simulink model "D53_LKA_Software"  (R2018b)
settings: Solver=ode3  StartTime=0.0  StopTime=10.0  FixedStep=0.01  RelTol=1e-3  EnableMultiTasking=on
model workspace (MAT data in the model file):
  MCOS : class17 (value not decoded)
  MCOS : class17 (value not decoded)
  MCOS : class17 (value not decoded)
  MCOS : class17 (value not decoded)
  MCOS : class17 (value not decoded)
  MCOS : class17 (value not decoded)
  MCOS : class17 (value not decoded)
  MCOS : class17 (value not decoded)
  MCOS : class17 (value not decoded)
  MCOS : class17 (value not decoded)
  MCOS : class17 (value not decoded)
  MCOS : class17 (value not decoded)
  MCOS : class17 (value not decoded)
  MCOS : class17 (value not decoded)
  MCOS : class17 (value not decoded)
  MCOS : class17 (value not decoded)
  MCOS : class17 (value not decoded)
  MCOS : class17 (value not decoded)
  MCOS : class17 (value not decoded)
  MCOS : class17 (value not decoded)
  MCOS : class17 (value not decoded)
  MCOS : class17 (value not decoded)
  MCOS : class17 (value not decoded)
  MCOS : class17 (value not decoded)
  MCOS : class17 (value not decoded)
  MCOS : class17 (value not decoded)
  MCOS : class17 (value not decoded)
  MCOS : class17 (value not decoded)
  MCOS : class17 (value not decoded)
  MCOS : class17 (value not decoded)
  MCOS : class17 (value not decoded)
  MCOS : class17 (value not decoded)
  MCOS : class17 (value not decoded)
  MCOS : class17 (value not decoded)
  MCOS : class17 (value not decoded)
  MCOS : class17 (value not decoded)
  MCOS : class17 (value not decoded)
  MCOS : class17 (value not decoded)
  MCOS : class17 (value not decoded)
  MCOS : class17 (value not decoded)
  MCOS : class17 (value not decoded)
  MCOS : class17 (value not decoded)
  MCOS : class17 (value not decoded)
  MCOS : class17 (value not decoded)
  MCOS : class17 (value not decoded)
  MCOS : class17 (value not decoded)
  MCOS : class17 (value not decoded)
  MCOS : class17 (value not decoded)
  MCOS : class17 (value not decoded)
  MCOS : class17 (value not decoded)
  MCOS : class17 (value not decoded)
  MCOS : class17 (value not decoded)
  MCOS : class17 (value not decoded)
  MCOS : class17 (value not decoded)
  MCOS : class17 (value not decoded)
  MCOS : class17 (value not decoded)
  MCOS : class17 (value not decoded)
  MCOS : class17 (value not decoded)
  MCOS : class17 (value not decoded)
  MCOS : class17 (value not decoded)
  MCOS : class17 (value not decoded)
  MCOS : class17 (value not decoded)
  MCOS : class17 (value not decoded)
  MCOS : class17 (value not decoded)
  MCOS : class17 (value not decoded)
  MCOS : class17 (value not decoded)
  MCOS : class17 (value not decoded)
  MCOS : class17 (value not decoded)
  MCOS : class17 (value not decoded)
  MCOS : class17 (value not decoded)
  MCOS : class17 (value not decoded)
  MCOS : class17 (value not decoded)
  MCOS : class17 (value not decoded)
  MCOS : class17 (value not decoded)
  MCOS : class17 (value not decoded)
  MCOS : class17 (value not decoded)
  MCOS : class17 (value not decoded)
  MCOS : class17 (value not decoded)
  MCOS : class17 (value not decoded)
  MCOS : class17 (value not decoded)
  MCOS : class17 (value not decoded)
  MCOS : class17 (value not decoded)
  MCOS : class17 (value not decoded)
  MCOS : class17 (value not decoded)
  MCOS : class17 (value not decoded)
  MCOS : class17 (value not decoded)
  MCOS : class17 (value not decoded)
  MCOS : class17 (value not decoded)
  MCOS : class17 (value not decoded)
undefined symbols (not defined in the file or in its folder): LKA_CarWidth, LKA_SampleTime, LKA_StrRatio_C, LKA_Veh2CamL_C, LKA_Veh2CamW_C, LKA_WhlBaseL_C, LL_CompSWA_C, LL_CrvtPrvwT_C, LL_DesDvt_C, LL_DvtComp_C, LL_DvtPrvwT_C, LL_DvtSpdDet_vDvtSpdMin_C, LL_HdAgExT_C, LL_HdAgPrvwT_C, LL_LAccMax_C, LL_LAccRMax_C, LL_LDW_EarliestWarnLine_C, LL_LDW_LatestWarnLine_C, LL_LDWS_SUPPRESS_HEADING, LL_LFClb_TFC_DiffCtlBalance, LL_LFClb_TFC_DiffCtrlMaxSWA, LL_LFClb_TFC_DiffCtrlRatio, LL_LFClb_TFC_facmGainLutGain1_C, LL_LFClb_TFC_facmGainLutGain2_C, LL_LFClb_TFC_facmIntegRatio, LL_LFClb_TFC_facmKlat_C, LL_LFClb_TFC_FfCtlRatio_C, LL_LFClb_TFC_phiIntegCtlMaxSWA_C, LL_LFClb_TFC_tiKlatPrvwT_C, LL_LFClb_TFC_vGainLutVehSpdLwr_C, LL_LFClb_TFC_vGainLutVehSpdUpr_C, LL_LKA_EarliestWarnLine_C, LL_LKA_LatestWarnLine_C, LL_LKAExPrcs_ExitC0Dvt, LL_LKAExPrcs_ExitC0Swt, LL_LKAExPrcs_tiExitTime1, LL_LKAExPrcs_tiExitTime2, LL_LKAExPrcs_tiExitTime3, LL_LKAS_OUT_OF_CONTROL_LAT_VEL, LL_LKAS_OUT_OF_CONTROL_TTLC, LL_LKASWASyn_M0, LL_LKASWASyn_M1, LL_LKASWASyn_M2, LL_LKASWASyn_M3K, LL_LKASWASyn_SWAaddMax, LL_LKASWASyn_T2, LL_LKASWASyn_tiTrqSwaRtTime, LL_LKASWASyn_tiTrqSwaTime, LL_LKASWASyn_TrqMax, LL_LKASWASyn_TrqSwaAddSwt, LL_LKASWASyn_TrqSwaRateDiff, LL_LSpdCompT_C, LL_lStpLngth_C, LL_MAX_DELAY_EPSSTAR_TIME, LL_MAX_DRIVER_TORQUE_DISABLE, LL_MAX_DRIVER_TORQUE_ENABLE, LL_MAX_LANE_WIDTH_DISABLE, LL_MAX_LANE_WIDTH_ENABLE, LL_MAX_LAT_ACC_DISABLE, LL_MAX_LAT_ACC_ENABLE ... (+30)
libraries: simulink x167, canmsglib x52, dspstat3 x3, simulink_extras x1
(part 20 of 21)

== system D53_LKA_Software/SignalBusCreator/Body Electric System State Receive and Processing (BESRx)/Steering Lamp CAN Frame PreProcess (StLampCANFrmPPrcs)/CAN Diagnosis (CANDia)/CheckSum Diagnosis (ChkSumDia)/Bit Check(BChk)/Bit Operating (BOp)/ChksumPre7 ==
  In1 : Inport
  Data Type Conversion8 : DataTypeConversion  OutDataTypeStr=uint16
  Extract Bits1 : simulink/Logic and Bit Operations/Extract Bits  bitsToExtract=Range of bits  numBits=8  bitIdxRange=7  outScalingMode=Treat bit field as an integer
      settings: SourceProductName=Simulink
  Out1 : Outport
  wires:
  Data Type Conversion8/1 -> Out1/1
  In1/1 -> Extract Bits1/1
  Extract Bits1/1 -> Data Type Conversion8/1

== system D53_LKA_Software/SignalBusCreator/Function Keys State Receive and Processing (FKeyStRx)/Key Enable CAN Frame PreProcess (KeyEnaCANFrmPPrcs)/CAN Diagnosis (CANDia)/CheckSum Diagnosis (ChkSumDia)/Bit Check(BChk)/Bit Operating (BOp)/ChksumPre1 ==
  In1 : Inport
  Data Type Conversion7 : DataTypeConversion  OutDataTypeStr=uint16
  Out1 : Outport
  wires:
  Data Type Conversion7/1 -> Out1/1
  In1/1 -> Data Type Conversion7/1

== system D53_LKA_Software/SignalBusCreator/Function Keys State Receive and Processing (FKeyStRx)/Key Enable CAN Frame PreProcess (KeyEnaCANFrmPPrcs)/CAN Diagnosis (CANDia)/CheckSum Diagnosis (ChkSumDia)/Bit Check(BChk)/Bit Operating (BOp)/ChksumPre2 ==
  In1 : Inport
  Data Type Conversion7 : DataTypeConversion  OutDataTypeStr=uint16
  Extract Bits : simulink/Logic and Bit Operations/Extract Bits  bitsToExtract=Range of bits  numBits=8  bitIdxRange=6  outScalingMode=Treat bit field as an integer
      settings: SourceProductName=Simulink
  Out1 : Outport
  wires:
  Extract Bits/1 -> Data Type Conversion7/1
  In1/1 -> Extract Bits/1
  Data Type Conversion7/1 -> Out1/1

== system D53_LKA_Software/SignalBusCreator/Function Keys State Receive and Processing (FKeyStRx)/Key Enable CAN Frame PreProcess (KeyEnaCANFrmPPrcs)/CAN Diagnosis (CANDia)/CheckSum Diagnosis (ChkSumDia)/Bit Check(BChk)/Bit Operating (BOp)/ChksumPre3 ==
  In1 : Inport
  Data Type Conversion8 : DataTypeConversion  OutDataTypeStr=uint16
  Extract Bits1 : simulink/Logic and Bit Operations/Extract Bits  bitsToExtract=Range of bits  numBits=8  bitIdxRange=5  outScalingMode=Treat bit field as an integer
      settings: SourceProductName=Simulink
  Out1 : Outport
  wires:
  Extract Bits1/1 -> Data Type Conversion8/1
  In1/1 -> Extract Bits1/1
  Data Type Conversion8/1 -> Out1/1

== system D53_LKA_Software/SignalBusCreator/Function Keys State Receive and Processing (FKeyStRx)/Key Enable CAN Frame PreProcess (KeyEnaCANFrmPPrcs)/CAN Diagnosis (CANDia)/CheckSum Diagnosis (ChkSumDia)/Bit Check(BChk)/Bit Operating (BOp)/ChksumPre4 ==
  In1 : Inport
  Data Type Conversion8 : DataTypeConversion  OutDataTypeStr=uint16
  Extract Bits1 : simulink/Logic and Bit Operations/Extract Bits  bitsToExtract=Range of bits  numBits=8  bitIdxRange=4  outScalingMode=Treat bit field as an integer
      settings: SourceProductName=Simulink
  Out1 : Outport
  wires:
  Data Type Conversion8/1 -> Out1/1
  In1/1 -> Extract Bits1/1
  Extract Bits1/1 -> Data Type Conversion8/1

== system D53_LKA_Software/SignalBusCreator/Function Keys State Receive and Processing (FKeyStRx)/Key Enable CAN Frame PreProcess (KeyEnaCANFrmPPrcs)/CAN Diagnosis (CANDia)/CheckSum Diagnosis (ChkSumDia)/Bit Check(BChk)/Bit Operating (BOp)/ChksumPre5 ==
  In1 : Inport
  In2 : Inport  Port=2
  Add : Sum
  Data Type Conversion1 : DataTypeConversion  OutDataTypeStr=uint16
  Data Type Conversion4 : DataTypeConversion  OutDataTypeStr=uint16
  Shift Arithmetic2 : ArithShift  BitShiftNumber=-8
  Out1 : Outport
  wires:
  Data Type Conversion1/1 -> Add/2
  Data Type Conversion4/1 -> Shift Arithmetic2/1
  Add/1 -> Out1/1
  Shift Arithmetic2/1 -> Add/1
  In2/1 -> Data Type Conversion1/1
  In1/1 -> Data Type Conversion4/1

== system D53_LKA_Software/SignalBusCreator/Function Keys State Receive and Processing (FKeyStRx)/Key Enable CAN Frame PreProcess (KeyEnaCANFrmPPrcs)/CAN Diagnosis (CANDia)/CheckSum Diagnosis (ChkSumDia)/Bit Check(BChk)/Bit Operating (BOp)/ChksumPre6 ==
  In1 : Inport
  In2 : Inport  Port=2
  Add : Sum
  Data Type Conversion1 : DataTypeConversion  OutDataTypeStr=uint16
  Data Type Conversion4 : DataTypeConversion  OutDataTypeStr=uint16
  Shift Arithmetic2 : ArithShift  BitShiftNumber=-8
  Out1 : Outport
  wires:
  In1/1 -> Data Type Conversion4/1
  In2/1 -> Data Type Conversion1/1
  Shift Arithmetic2/1 -> Add/1
  Add/1 -> Out1/1
  Data Type Conversion4/1 -> Shift Arithmetic2/1
  Data Type Conversion1/1 -> Add/2

== system D53_LKA_Software/SignalBusCreator/Function Keys State Receive and Processing (FKeyStRx)/Key Enable CAN Frame PreProcess (KeyEnaCANFrmPPrcs)/CAN Diagnosis (CANDia)/CheckSum Diagnosis (ChkSumDia)/Bit Check(BChk)/Bit Operating (BOp)/ChksumPre7 ==
  In1 : Inport
  Data Type Conversion8 : DataTypeConversion  OutDataTypeStr=uint16
  Extract Bits1 : simulink/Logic and Bit Operations/Extract Bits  bitsToExtract=Range of bits  numBits=8  bitIdxRange=7  outScalingMode=Treat bit field as an integer
      settings: SourceProductName=Simulink
  Out1 : Outport
  wires:
  Extract Bits1/1 -> Data Type Conversion8/1
  In1/1 -> Extract Bits1/1
  Data Type Conversion8/1 -> Out1/1

== system D53_LKA_Software/SignalBusCreator/Lanes Information Receive and Processing (LaneRx)/L0 Information (L0Info) /CAN Diagnosis (CANDia)/CheckSum Diagnosis (ChkSumDia)/Bit Check(BChk)/Bit Operating (BOp)/ChksumPre1 ==
  In1 : Inport
  Data Type Conversion7 : DataTypeConversion  OutDataTypeStr=uint16
  Out1 : Outport
  wires:
  In1/1 -> Data Type Conversion7/1
  Data Type Conversion7/1 -> Out1/1

== system D53_LKA_Software/SignalBusCreator/Lanes Information Receive and Processing (LaneRx)/L0 Information (L0Info) /CAN Diagnosis (CANDia)/CheckSum Diagnosis (ChkSumDia)/Bit Check(BChk)/Bit Operating (BOp)/ChksumPre2 ==
  In1 : Inport
  Data Type Conversion7 : DataTypeConversion  OutDataTypeStr=uint16
  Extract Bits : simulink/Logic and Bit Operations/Extract Bits  bitsToExtract=Range of bits  numBits=8  bitIdxRange=6  outScalingMode=Treat bit field as an integer
      settings: SourceProductName=Simulink
  Out1 : Outport
  wires:
  Data Type Conversion7/1 -> Out1/1
  In1/1 -> Extract Bits/1
  Extract Bits/1 -> Data Type Conversion7/1

== system D53_LKA_Software/SignalBusCreator/Lanes Information Receive and Processing (LaneRx)/L0 Information (L0Info) /CAN Diagnosis (CANDia)/CheckSum Diagnosis (ChkSumDia)/Bit Check(BChk)/Bit Operating (BOp)/ChksumPre3 ==
  In1 : Inport
  Data Type Conversion8 : DataTypeConversion  OutDataTypeStr=uint16
  Extract Bits1 : simulink/Logic and Bit Operations/Extract Bits  bitsToExtract=Range of bits  numBits=8  bitIdxRange=5  outScalingMode=Treat bit field as an integer
      settings: SourceProductName=Simulink
  Out1 : Outport
  wires:
  Data Type Conversion8/1 -> Out1/1
  In1/1 -> Extract Bits1/1
  Extract Bits1/1 -> Data Type Conversion8/1

== system D53_LKA_Software/SignalBusCreator/Lanes Information Receive and Processing (LaneRx)/L0 Information (L0Info) /CAN Diagnosis (CANDia)/CheckSum Diagnosis (ChkSumDia)/Bit Check(BChk)/Bit Operating (BOp)/ChksumPre4 ==
  In1 : Inport
  Data Type Conversion8 : DataTypeConversion  OutDataTypeStr=uint16
  Extract Bits1 : simulink/Logic and Bit Operations/Extract Bits  bitsToExtract=Range of bits  numBits=8  bitIdxRange=4  outScalingMode=Treat bit field as an integer
      settings: SourceProductName=Simulink
  Out1 : Outport
  wires:
  Extract Bits1/1 -> Data Type Conversion8/1
  In1/1 -> Extract Bits1/1
  Data Type Conversion8/1 -> Out1/1

== system D53_LKA_Software/SignalBusCreator/Lanes Information Receive and Processing (LaneRx)/L0 Information (L0Info) /CAN Diagnosis (CANDia)/CheckSum Diagnosis (ChkSumDia)/Bit Check(BChk)/Bit Operating (BOp)/ChksumPre5 ==
  In1 : Inport
  In2 : Inport  Port=2
  Add : Sum
  Data Type Conversion1 : DataTypeConversion  OutDataTypeStr=uint16
  Data Type Conversion4 : DataTypeConversion  OutDataTypeStr=uint16
  Shift Arithmetic2 : ArithShift  BitShiftNumber=-8
  Out1 : Outport
  wires:
  In1/1 -> Data Type Conversion4/1
  In2/1 -> Data Type Conversion1/1
  Shift Arithmetic2/1 -> Add/1
  Add/1 -> Out1/1
  Data Type Conversion4/1 -> Shift Arithmetic2/1
  Data Type Conversion1/1 -> Add/2

== system D53_LKA_Software/SignalBusCreator/Lanes Information Receive and Processing (LaneRx)/L0 Information (L0Info) /CAN Diagnosis (CANDia)/CheckSum Diagnosis (ChkSumDia)/Bit Check(BChk)/Bit Operating (BOp)/ChksumPre6 ==
  In1 : Inport
  In2 : Inport  Port=2
  Add : Sum
  Data Type Conversion1 : DataTypeConversion  OutDataTypeStr=uint16
  Data Type Conversion4 : DataTypeConversion  OutDataTypeStr=uint16
  Shift Arithmetic2 : ArithShift  BitShiftNumber=-8
  Out1 : Outport
  wires:
  Data Type Conversion1/1 -> Add/2
  Data Type Conversion4/1 -> Shift Arithmetic2/1
  Add/1 -> Out1/1
  Shift Arithmetic2/1 -> Add/1
  In2/1 -> Data Type Conversion1/1
  In1/1 -> Data Type Conversion4/1

== system D53_LKA_Software/SignalBusCreator/Lanes Information Receive and Processing (LaneRx)/L0 Information (L0Info) /CAN Diagnosis (CANDia)/CheckSum Diagnosis (ChkSumDia)/Bit Check(BChk)/Bit Operating (BOp)/ChksumPre7 ==
  In1 : Inport
  Data Type Conversion8 : DataTypeConversion  OutDataTypeStr=uint16
  Extract Bits1 : simulink/Logic and Bit Operations/Extract Bits  bitsToExtract=Range of bits  numBits=8  bitIdxRange=7  outScalingMode=Treat bit field as an integer
      settings: SourceProductName=Simulink
  Out1 : Outport
  wires:
  Data Type Conversion8/1 -> Out1/1
  In1/1 -> Extract Bits1/1
  Extract Bits1/1 -> Data Type Conversion8/1

== system D53_LKA_Software/SignalBusCreator/Lanes Information Receive and Processing (LaneRx)/L1 Information (L1Info)/CAN Diagnosis (CANDia)/CheckSum Diagnosis (ChkSumDia)/Bit Check(BChk)/Bit Operating (BOp)/ChksumPre1 ==
  In1 : Inport
  Data Type Conversion7 : DataTypeConversion  OutDataTypeStr=uint16
  Out1 : Outport
  wires:
  Data Type Conversion7/1 -> Out1/1
  In1/1 -> Data Type Conversion7/1

== system D53_LKA_Software/SignalBusCreator/Lanes Information Receive and Processing (LaneRx)/L1 Information (L1Info)/CAN Diagnosis (CANDia)/CheckSum Diagnosis (ChkSumDia)/Bit Check(BChk)/Bit Operating (BOp)/ChksumPre2 ==
  In1 : Inport
  Data Type Conversion7 : DataTypeConversion  OutDataTypeStr=uint16
  Extract Bits : simulink/Logic and Bit Operations/Extract Bits  bitsToExtract=Range of bits  numBits=8  bitIdxRange=6  outScalingMode=Treat bit field as an integer
      settings: SourceProductName=Simulink
  Out1 : Outport
  wires:
  Extract Bits/1 -> Data Type Conversion7/1
  In1/1 -> Extract Bits/1
  Data Type Conversion7/1 -> Out1/1

== system D53_LKA_Software/SignalBusCreator/Lanes Information Receive and Processing (LaneRx)/L1 Information (L1Info)/CAN Diagnosis (CANDia)/CheckSum Diagnosis (ChkSumDia)/Bit Check(BChk)/Bit Operating (BOp)/ChksumPre3 ==
  In1 : Inport
  Data Type Conversion8 : DataTypeConversion  OutDataTypeStr=uint16
  Extract Bits1 : simulink/Logic and Bit Operations/Extract Bits  bitsToExtract=Range of bits  numBits=8  bitIdxRange=5  outScalingMode=Treat bit field as an integer
      settings: SourceProductName=Simulink
  Out1 : Outport
  wires:
  Extract Bits1/1 -> Data Type Conversion8/1
  In1/1 -> Extract Bits1/1
  Data Type Conversion8/1 -> Out1/1

== system D53_LKA_Software/SignalBusCreator/Lanes Information Receive and Processing (LaneRx)/L1 Information (L1Info)/CAN Diagnosis (CANDia)/CheckSum Diagnosis (ChkSumDia)/Bit Check(BChk)/Bit Operating (BOp)/ChksumPre4 ==
  In1 : Inport
  Data Type Conversion8 : DataTypeConversion  OutDataTypeStr=uint16
  Extract Bits1 : simulink/Logic and Bit Operations/Extract Bits  bitsToExtract=Range of bits  numBits=8  bitIdxRange=4  outScalingMode=Treat bit field as an integer
      settings: SourceProductName=Simulink
  Out1 : Outport
  wires:
  Data Type Conversion8/1 -> Out1/1
  In1/1 -> Extract Bits1/1
  Extract Bits1/1 -> Data Type Conversion8/1

== system D53_LKA_Software/SignalBusCreator/Lanes Information Receive and Processing (LaneRx)/L1 Information (L1Info)/CAN Diagnosis (CANDia)/CheckSum Diagnosis (ChkSumDia)/Bit Check(BChk)/Bit Operating (BOp)/ChksumPre5 ==
  In1 : Inport
  In2 : Inport  Port=2
  Add : Sum
  Data Type Conversion1 : DataTypeConversion  OutDataTypeStr=uint16
  Data Type Conversion4 : DataTypeConversion  OutDataTypeStr=uint16
  Shift Arithmetic2 : ArithShift  BitShiftNumber=-8
  Out1 : Outport
  wires:
  Data Type Conversion1/1 -> Add/2
  Data Type Conversion4/1 -> Shift Arithmetic2/1
  Add/1 -> Out1/1
  Shift Arithmetic2/1 -> Add/1
  In2/1 -> Data Type Conversion1/1
  In1/1 -> Data Type Conversion4/1

== system D53_LKA_Software/SignalBusCreator/Lanes Information Receive and Processing (LaneRx)/L1 Information (L1Info)/CAN Diagnosis (CANDia)/CheckSum Diagnosis (ChkSumDia)/Bit Check(BChk)/Bit Operating (BOp)/ChksumPre6 ==
  In1 : Inport
  In2 : Inport  Port=2
  Add : Sum
  Data Type Conversion1 : DataTypeConversion  OutDataTypeStr=uint16
  Data Type Conversion4 : DataTypeConversion  OutDataTypeStr=uint16
  Shift Arithmetic2 : ArithShift  BitShiftNumber=-8
  Out1 : Outport
  wires:
  In1/1 -> Data Type Conversion4/1
  In2/1 -> Data Type Conversion1/1
  Shift Arithmetic2/1 -> Add/1
  Add/1 -> Out1/1
  Data Type Conversion4/1 -> Shift Arithmetic2/1
  Data Type Conversion1/1 -> Add/2

== system D53_LKA_Software/SignalBusCreator/Lanes Information Receive and Processing (LaneRx)/L1 Information (L1Info)/CAN Diagnosis (CANDia)/CheckSum Diagnosis (ChkSumDia)/Bit Check(BChk)/Bit Operating (BOp)/ChksumPre7 ==
  In1 : Inport
  Data Type Conversion8 : DataTypeConversion  OutDataTypeStr=uint16
  Extract Bits1 : simulink/Logic and Bit Operations/Extract Bits  bitsToExtract=Range of bits  numBits=8  bitIdxRange=7  outScalingMode=Treat bit field as an integer
      settings: SourceProductName=Simulink
  Out1 : Outport
  wires:
  Extract Bits1/1 -> Data Type Conversion8/1
  In1/1 -> Extract Bits1/1
  Data Type Conversion8/1 -> Out1/1

== system D53_LKA_Software/SignalBusCreator/Lanes Information Receive and Processing (LaneRx)/R0 Information (R0Info)/CAN Diagnosis (CANDia)/CheckSum Diagnosis (ChkSumDia)/Bit Check(BChk)/Bit Operating (BOp)/ChksumPre1 ==
  In1 : Inport
  Data Type Conversion7 : DataTypeConversion  OutDataTypeStr=uint16
  Out1 : Outport
  wires:
  Data Type Conversion7/1 -> Out1/1
  In1/1 -> Data Type Conversion7/1

== system D53_LKA_Software/SignalBusCreator/Lanes Information Receive and Processing (LaneRx)/R0 Information (R0Info)/CAN Diagnosis (CANDia)/CheckSum Diagnosis (ChkSumDia)/Bit Check(BChk)/Bit Operating (BOp)/ChksumPre2 ==
  In1 : Inport
  Data Type Conversion7 : DataTypeConversion  OutDataTypeStr=uint16
  Extract Bits : simulink/Logic and Bit Operations/Extract Bits  bitsToExtract=Range of bits  numBits=8  bitIdxRange=6  outScalingMode=Treat bit field as an integer
      settings: SourceProductName=Simulink
  Out1 : Outport
  wires:
  Extract Bits/1 -> Data Type Conversion7/1
  In1/1 -> Extract Bits/1
  Data Type Conversion7/1 -> Out1/1

== system D53_LKA_Software/SignalBusCreator/Lanes Information Receive and Processing (LaneRx)/R0 Information (R0Info)/CAN Diagnosis (CANDia)/CheckSum Diagnosis (ChkSumDia)/Bit Check(BChk)/Bit Operating (BOp)/ChksumPre3 ==
  In1 : Inport
  Data Type Conversion8 : DataTypeConversion  OutDataTypeStr=uint16
  Extract Bits1 : simulink/Logic and Bit Operations/Extract Bits  bitsToExtract=Range of bits  numBits=8  bitIdxRange=5  outScalingMode=Treat bit field as an integer
      settings: SourceProductName=Simulink
  Out1 : Outport
  wires:
  Extract Bits1/1 -> Data Type Conversion8/1
  In1/1 -> Extract Bits1/1
  Data Type Conversion8/1 -> Out1/1

== system D53_LKA_Software/SignalBusCreator/Lanes Information Receive and Processing (LaneRx)/R0 Information (R0Info)/CAN Diagnosis (CANDia)/CheckSum Diagnosis (ChkSumDia)/Bit Check(BChk)/Bit Operating (BOp)/ChksumPre4 ==
  In1 : Inport
  Data Type Conversion8 : DataTypeConversion  OutDataTypeStr=uint16
  Extract Bits1 : simulink/Logic and Bit Operations/Extract Bits  bitsToExtract=Range of bits  numBits=8  bitIdxRange=4  outScalingMode=Treat bit field as an integer
      settings: SourceProductName=Simulink
  Out1 : Outport
  wires:
  Data Type Conversion8/1 -> Out1/1
  In1/1 -> Extract Bits1/1
  Extract Bits1/1 -> Data Type Conversion8/1

== system D53_LKA_Software/SignalBusCreator/Lanes Information Receive and Processing (LaneRx)/R0 Information (R0Info)/CAN Diagnosis (CANDia)/CheckSum Diagnosis (ChkSumDia)/Bit Check(BChk)/Bit Operating (BOp)/ChksumPre5 ==
  In1 : Inport
  In2 : Inport  Port=2
  Add : Sum
  Data Type Conversion1 : DataTypeConversion  OutDataTypeStr=uint16
  Data Type Conversion4 : DataTypeConversion  OutDataTypeStr=uint16
  Shift Arithmetic2 : ArithShift  BitShiftNumber=-8
  Out1 : Outport
  wires:
  Data Type Conversion1/1 -> Add/2
  Data Type Conversion4/1 -> Shift Arithmetic2/1
  Add/1 -> Out1/1
  Shift Arithmetic2/1 -> Add/1
  In2/1 -> Data Type Conversion1/1
  In1/1 -> Data Type Conversion4/1

== system D53_LKA_Software/SignalBusCreator/Lanes Information Receive and Processing (LaneRx)/R0 Information (R0Info)/CAN Diagnosis (CANDia)/CheckSum Diagnosis (ChkSumDia)/Bit Check(BChk)/Bit Operating (BOp)/ChksumPre6 ==
  In1 : Inport
  In2 : Inport  Port=2
  Add : Sum
  Data Type Conversion1 : DataTypeConversion  OutDataTypeStr=uint16
  Data Type Conversion4 : DataTypeConversion  OutDataTypeStr=uint16
  Shift Arithmetic2 : ArithShift  BitShiftNumber=-8
  Out1 : Outport
  wires:
  In1/1 -> Data Type Conversion4/1
  In2/1 -> Data Type Conversion1/1
  Shift Arithmetic2/1 -> Add/1
  Add/1 -> Out1/1
  Data Type Conversion4/1 -> Shift Arithmetic2/1
  Data Type Conversion1/1 -> Add/2

== system D53_LKA_Software/SignalBusCreator/Lanes Information Receive and Processing (LaneRx)/R0 Information (R0Info)/CAN Diagnosis (CANDia)/CheckSum Diagnosis (ChkSumDia)/Bit Check(BChk)/Bit Operating (BOp)/ChksumPre7 ==
  In1 : Inport
  Data Type Conversion8 : DataTypeConversion  OutDataTypeStr=uint16
  Extract Bits1 : simulink/Logic and Bit Operations/Extract Bits  bitsToExtract=Range of bits  numBits=8  bitIdxRange=7  outScalingMode=Treat bit field as an integer
      settings: SourceProductName=Simulink
  Out1 : Outport
  wires:
  Extract Bits1/1 -> Data Type Conversion8/1
  In1/1 -> Extract Bits1/1
  Data Type Conversion8/1 -> Out1/1

== system D53_LKA_Software/SignalBusCreator/Lanes Information Receive and Processing (LaneRx)/R1 Information (R1Info)/CAN Diagnosis (CANDia)/CheckSum Diagnosis (ChkSumDia)/Bit Check(BChk)/Bit Operating (BOp)/ChksumPre1 ==
  In1 : Inport
  Data Type Conversion7 : DataTypeConversion  OutDataTypeStr=uint16
  Out1 : Outport
  wires:
  In1/1 -> Data Type Conversion7/1
  Data Type Conversion7/1 -> Out1/1

== system D53_LKA_Software/SignalBusCreator/Lanes Information Receive and Processing (LaneRx)/R1 Information (R1Info)/CAN Diagnosis (CANDia)/CheckSum Diagnosis (ChkSumDia)/Bit Check(BChk)/Bit Operating (BOp)/ChksumPre2 ==
  In1 : Inport
  Data Type Conversion7 : DataTypeConversion  OutDataTypeStr=uint16
  Extract Bits : simulink/Logic and Bit Operations/Extract Bits  bitsToExtract=Range of bits  numBits=8  bitIdxRange=6  outScalingMode=Treat bit field as an integer
      settings: SourceProductName=Simulink
  Out1 : Outport
  wires:
  Data Type Conversion7/1 -> Out1/1
  In1/1 -> Extract Bits/1
  Extract Bits/1 -> Data Type Conversion7/1

== system D53_LKA_Software/SignalBusCreator/Lanes Information Receive and Processing (LaneRx)/R1 Information (R1Info)/CAN Diagnosis (CANDia)/CheckSum Diagnosis (ChkSumDia)/Bit Check(BChk)/Bit Operating (BOp)/ChksumPre3 ==
  In1 : Inport
  Data Type Conversion8 : DataTypeConversion  OutDataTypeStr=uint16
  Extract Bits1 : simulink/Logic and Bit Operations/Extract Bits  bitsToExtract=Range of bits  numBits=8  bitIdxRange=5  outScalingMode=Treat bit field as an integer
      settings: SourceProductName=Simulink
  Out1 : Outport
  wires:
  Data Type Conversion8/1 -> Out1/1
  In1/1 -> Extract Bits1/1
  Extract Bits1/1 -> Data Type Conversion8/1

== system D53_LKA_Software/SignalBusCreator/Lanes Information Receive and Processing (LaneRx)/R1 Information (R1Info)/CAN Diagnosis (CANDia)/CheckSum Diagnosis (ChkSumDia)/Bit Check(BChk)/Bit Operating (BOp)/ChksumPre4 ==
  In1 : Inport
  Data Type Conversion8 : DataTypeConversion  OutDataTypeStr=uint16
  Extract Bits1 : simulink/Logic and Bit Operations/Extract Bits  bitsToExtract=Range of bits  numBits=8  bitIdxRange=4  outScalingMode=Treat bit field as an integer
      settings: SourceProductName=Simulink
  Out1 : Outport
  wires:
  Extract Bits1/1 -> Data Type Conversion8/1
  In1/1 -> Extract Bits1/1
  Data Type Conversion8/1 -> Out1/1

== system D53_LKA_Software/SignalBusCreator/Lanes Information Receive and Processing (LaneRx)/R1 Information (R1Info)/CAN Diagnosis (CANDia)/CheckSum Diagnosis (ChkSumDia)/Bit Check(BChk)/Bit Operating (BOp)/ChksumPre5 ==
  In1 : Inport
  In2 : Inport  Port=2
  Add : Sum
  Data Type Conversion1 : DataTypeConversion  OutDataTypeStr=uint16
  Data Type Conversion4 : DataTypeConversion  OutDataTypeStr=uint16
  Shift Arithmetic2 : ArithShift  BitShiftNumber=-8
  Out1 : Outport
  wires:
  In1/1 -> Data Type Conversion4/1
  In2/1 -> Data Type Conversion1/1
  Shift Arithmetic2/1 -> Add/1
  Add/1 -> Out1/1
  Data Type Conversion4/1 -> Shift Arithmetic2/1
  Data Type Conversion1/1 -> Add/2

== system D53_LKA_Software/SignalBusCreator/Lanes Information Receive and Processing (LaneRx)/R1 Information (R1Info)/CAN Diagnosis (CANDia)/CheckSum Diagnosis (ChkSumDia)/Bit Check(BChk)/Bit Operating (BOp)/ChksumPre6 ==
  In1 : Inport
  In2 : Inport  Port=2
  Add : Sum
  Data Type Conversion1 : DataTypeConversion  OutDataTypeStr=uint16
  Data Type Conversion4 : DataTypeConversion  OutDataTypeStr=uint16
  Shift Arithmetic2 : ArithShift  BitShiftNumber=-8
  Out1 : Outport
  wires:
  Data Type Conversion1/1 -> Add/2
  Data Type Conversion4/1 -> Shift Arithmetic2/1
  Add/1 -> Out1/1
  Shift Arithmetic2/1 -> Add/1
  In2/1 -> Data Type Conversion1/1
  In1/1 -> Data Type Conversion4/1

== system D53_LKA_Software/SignalBusCreator/Lanes Information Receive and Processing (LaneRx)/R1 Information (R1Info)/CAN Diagnosis (CANDia)/CheckSum Diagnosis (ChkSumDia)/Bit Check(BChk)/Bit Operating (BOp)/ChksumPre7 ==
  In1 : Inport
  Data Type Conversion8 : DataTypeConversion  OutDataTypeStr=uint16
  Extract Bits1 : simulink/Logic and Bit Operations/Extract Bits  bitsToExtract=Range of bits  numBits=8  bitIdxRange=7  outScalingMode=Treat bit field as an integer
      settings: SourceProductName=Simulink
  Out1 : Outport
  wires:
  Data Type Conversion8/1 -> Out1/1
  In1/1 -> Extract Bits1/1
  Extract Bits1/1 -> Data Type Conversion8/1

== system D53_LKA_Software/SignalBusCreator/Vehicle Movement Signal Receive and Processing (VehMovRx)/VehSpd CAN Frame PreProcess (VehSpdCANFrmPPrcs)/CAN Diagnosis (CANDia)/CheckSum Diagnosis (ChkSumDia)/Bit Check(BChk)/Bit Operating (BOp)/ChksumPre1 ==
  In1 : Inport
  Data Type Conversion7 : DataTypeConversion  OutDataTypeStr=uint16
  Out1 : Outport
  wires:
  Data Type Conversion7/1 -> Out1/1
  In1/1 -> Data Type Conversion7/1

== system D53_LKA_Software/SignalBusCreator/Vehicle Movement Signal Receive and Processing (VehMovRx)/VehSpd CAN Frame PreProcess (VehSpdCANFrmPPrcs)/CAN Diagnosis (CANDia)/CheckSum Diagnosis (ChkSumDia)/Bit Check(BChk)/Bit Operating (BOp)/ChksumPre2 ==
  In1 : Inport
  Data Type Conversion7 : DataTypeConversion  OutDataTypeStr=uint16
  Extract Bits : simulink/Logic and Bit Operations/Extract Bits  bitsToExtract=Range of bits  numBits=8  bitIdxRange=6  outScalingMode=Treat bit field as an integer
      settings: SourceProductName=Simulink
  Out1 : Outport
  wires:
  Extract Bits/1 -> Data Type Conversion7/1
  In1/1 -> Extract Bits/1
  Data Type Conversion7/1 -> Out1/1

== system D53_LKA_Software/SignalBusCreator/Vehicle Movement Signal Receive and Processing (VehMovRx)/VehSpd CAN Frame PreProcess (VehSpdCANFrmPPrcs)/CAN Diagnosis (CANDia)/CheckSum Diagnosis (ChkSumDia)/Bit Check(BChk)/Bit Operating (BOp)/ChksumPre3 ==
  In1 : Inport
  Data Type Conversion8 : DataTypeConversion  OutDataTypeStr=uint16
  Extract Bits1 : simulink/Logic and Bit Operations/Extract Bits  bitsToExtract=Range of bits  numBits=8  bitIdxRange=5  outScalingMode=Treat bit field as an integer
      settings: SourceProductName=Simulink
  Out1 : Outport
  wires:
  Extract Bits1/1 -> Data Type Conversion8/1
  In1/1 -> Extract Bits1/1
  Data Type Conversion8/1 -> Out1/1

== system D53_LKA_Software/SignalBusCreator/Vehicle Movement Signal Receive and Processing (VehMovRx)/VehSpd CAN Frame PreProcess (VehSpdCANFrmPPrcs)/CAN Diagnosis (CANDia)/CheckSum Diagnosis (ChkSumDia)/Bit Check(BChk)/Bit Operating (BOp)/ChksumPre4 ==
  In1 : Inport
  Data Type Conversion8 : DataTypeConversion  OutDataTypeStr=uint16
  Extract Bits1 : simulink/Logic and Bit Operations/Extract Bits  bitsToExtract=Range of bits  numBits=8  bitIdxRange=4  outScalingMode=Treat bit field as an integer
      settings: SourceProductName=Simulink
  Out1 : Outport
  wires:
  Data Type Conversion8/1 -> Out1/1
  In1/1 -> Extract Bits1/1
  Extract Bits1/1 -> Data Type Conversion8/1

== system D53_LKA_Software/SignalBusCreator/Vehicle Movement Signal Receive and Processing (VehMovRx)/VehSpd CAN Frame PreProcess (VehSpdCANFrmPPrcs)/CAN Diagnosis (CANDia)/CheckSum Diagnosis (ChkSumDia)/Bit Check(BChk)/Bit Operating (BOp)/ChksumPre5 ==
  In1 : Inport
  In2 : Inport  Port=2
  Add : Sum
  Data Type Conversion1 : DataTypeConversion  OutDataTypeStr=uint16
  Data Type Conversion4 : DataTypeConversion  OutDataTypeStr=uint16
  Shift Arithmetic2 : ArithShift  BitShiftNumber=-8
  Out1 : Outport
  wires:
  Data Type Conversion1/1 -> Add/2
  Data Type Conversion4/1 -> Shift Arithmetic2/1
  Add/1 -> Out1/1
  Shift Arithmetic2/1 -> Add/1
  In2/1 -> Data Type Conversion1/1
  In1/1 -> Data Type Conversion4/1

== system D53_LKA_Software/SignalBusCreator/Vehicle Movement Signal Receive and Processing (VehMovRx)/VehSpd CAN Frame PreProcess (VehSpdCANFrmPPrcs)/CAN Diagnosis (CANDia)/CheckSum Diagnosis (ChkSumDia)/Bit Check(BChk)/Bit Operating (BOp)/ChksumPre6 ==
  In1 : Inport
  In2 : Inport  Port=2
  Add : Sum
  Data Type Conversion1 : DataTypeConversion  OutDataTypeStr=uint16
  Data Type Conversion4 : DataTypeConversion  OutDataTypeStr=uint16
  Shift Arithmetic2 : ArithShift  BitShiftNumber=-8
  Out1 : Outport
  wires:
  In1/1 -> Data Type Conversion4/1
  In2/1 -> Data Type Conversion1/1
  Shift Arithmetic2/1 -> Add/1
  Add/1 -> Out1/1
  Data Type Conversion4/1 -> Shift Arithmetic2/1
  Data Type Conversion1/1 -> Add/2

== system D53_LKA_Software/SignalBusCreator/Vehicle Movement Signal Receive and Processing (VehMovRx)/VehSpd CAN Frame PreProcess (VehSpdCANFrmPPrcs)/CAN Diagnosis (CANDia)/CheckSum Diagnosis (ChkSumDia)/Bit Check(BChk)/Bit Operating (BOp)/ChksumPre7 ==
  In1 : Inport
  Data Type Conversion8 : DataTypeConversion  OutDataTypeStr=uint16
  Extract Bits1 : simulink/Logic and Bit Operations/Extract Bits  bitsToExtract=Range of bits  numBits=8  bitIdxRange=7  outScalingMode=Treat bit field as an integer
      settings: SourceProductName=Simulink
  Out1 : Outport
  wires:
  Extract Bits1/1 -> Data Type Conversion8/1
  In1/1 -> Extract Bits1/1
  Data Type Conversion8/1 -> Out1/1

== system D53_LKA_Software/SignalBusCreator/Vehicle Movement Signal Receive and Processing (VehMovRx)/Yaw State CAN Frame PreProcess (YawCANFrmPPrcs)/CAN Diagnosis (CANDia)/CheckSum Diagnosis (ChkSumDia)/Bit Check(BChk)/Bit Operating (BOp)/ChksumPre1 ==
  In1 : Inport
  Data Type Conversion7 : DataTypeConversion  OutDataTypeStr=uint16
  Out1 : Outport
  wires:
  Data Type Conversion7/1 -> Out1/1
  In1/1 -> Data Type Conversion7/1

== system D53_LKA_Software/SignalBusCreator/Vehicle Movement Signal Receive and Processing (VehMovRx)/Yaw State CAN Frame PreProcess (YawCANFrmPPrcs)/CAN Diagnosis (CANDia)/CheckSum Diagnosis (ChkSumDia)/Bit Check(BChk)/Bit Operating (BOp)/ChksumPre2 ==
  In1 : Inport
  Data Type Conversion7 : DataTypeConversion  OutDataTypeStr=uint16
  Extract Bits : simulink/Logic and Bit Operations/Extract Bits  bitsToExtract=Range of bits  numBits=8  bitIdxRange=6  outScalingMode=Treat bit field as an integer
      settings: SourceProductName=Simulink
  Out1 : Outport
  wires:
  Extract Bits/1 -> Data Type Conversion7/1
  In1/1 -> Extract Bits/1
  Data Type Conversion7/1 -> Out1/1

== system D53_LKA_Software/SignalBusCreator/Vehicle Movement Signal Receive and Processing (VehMovRx)/Yaw State CAN Frame PreProcess (YawCANFrmPPrcs)/CAN Diagnosis (CANDia)/CheckSum Diagnosis (ChkSumDia)/Bit Check(BChk)/Bit Operating (BOp)/ChksumPre3 ==
  In1 : Inport
  Data Type Conversion8 : DataTypeConversion  OutDataTypeStr=uint16
  Extract Bits1 : simulink/Logic and Bit Operations/Extract Bits  bitsToExtract=Range of bits  numBits=8  bitIdxRange=5  outScalingMode=Treat bit field as an integer
      settings: SourceProductName=Simulink
  Out1 : Outport
  wires:
  Extract Bits1/1 -> Data Type Conversion8/1
  In1/1 -> Extract Bits1/1
  Data Type Conversion8/1 -> Out1/1

== system D53_LKA_Software/SignalBusCreator/Vehicle Movement Signal Receive and Processing (VehMovRx)/Yaw State CAN Frame PreProcess (YawCANFrmPPrcs)/CAN Diagnosis (CANDia)/CheckSum Diagnosis (ChkSumDia)/Bit Check(BChk)/Bit Operating (BOp)/ChksumPre4 ==
  In1 : Inport
  Data Type Conversion8 : DataTypeConversion  OutDataTypeStr=uint16
  Extract Bits1 : simulink/Logic and Bit Operations/Extract Bits  bitsToExtract=Range of bits  numBits=8  bitIdxRange=4  outScalingMode=Treat bit field as an integer
      settings: SourceProductName=Simulink
  Out1 : Outport
  wires:
  Data Type Conversion8/1 -> Out1/1
  In1/1 -> Extract Bits1/1
  Extract Bits1/1 -> Data Type Conversion8/1

== system D53_LKA_Software/SignalBusCreator/Vehicle Movement Signal Receive and Processing (VehMovRx)/Yaw State CAN Frame PreProcess (YawCANFrmPPrcs)/CAN Diagnosis (CANDia)/CheckSum Diagnosis (ChkSumDia)/Bit Check(BChk)/Bit Operating (BOp)/ChksumPre5 ==
  In1 : Inport
  In2 : Inport  Port=2
  Add : Sum
  Data Type Conversion1 : DataTypeConversion  OutDataTypeStr=uint16
  Data Type Conversion4 : DataTypeConversion  OutDataTypeStr=uint16
  Shift Arithmetic2 : ArithShift  BitShiftNumber=-8
  Out1 : Outport
  wires:
  Data Type Conversion1/1 -> Add/2
  Data Type Conversion4/1 -> Shift Arithmetic2/1
  Add/1 -> Out1/1
  Shift Arithmetic2/1 -> Add/1
  In2/1 -> Data Type Conversion1/1
  In1/1 -> Data Type Conversion4/1

== system D53_LKA_Software/SignalBusCreator/Vehicle Movement Signal Receive and Processing (VehMovRx)/Yaw State CAN Frame PreProcess (YawCANFrmPPrcs)/CAN Diagnosis (CANDia)/CheckSum Diagnosis (ChkSumDia)/Bit Check(BChk)/Bit Operating (BOp)/ChksumPre6 ==
  In1 : Inport
  In2 : Inport  Port=2
  Add : Sum
  Data Type Conversion1 : DataTypeConversion  OutDataTypeStr=uint16
  Data Type Conversion4 : DataTypeConversion  OutDataTypeStr=uint16
  Shift Arithmetic2 : ArithShift  BitShiftNumber=-8
  Out1 : Outport
  wires:
  In1/1 -> Data Type Conversion4/1
  In2/1 -> Data Type Conversion1/1
  Shift Arithmetic2/1 -> Add/1
  Add/1 -> Out1/1
  Data Type Conversion4/1 -> Shift Arithmetic2/1
  Data Type Conversion1/1 -> Add/2

== system D53_LKA_Software/SignalBusCreator/Vehicle Movement Signal Receive and Processing (VehMovRx)/Yaw State CAN Frame PreProcess (YawCANFrmPPrcs)/CAN Diagnosis (CANDia)/CheckSum Diagnosis (ChkSumDia)/Bit Check(BChk)/Bit Operating (BOp)/ChksumPre7 ==
  In1 : Inport
  Data Type Conversion8 : DataTypeConversion  OutDataTypeStr=uint16
  Extract Bits1 : simulink/Logic and Bit Operations/Extract Bits  bitsToExtract=Range of bits  numBits=8  bitIdxRange=7  outScalingMode=Treat bit field as an integer
      settings: SourceProductName=Simulink
  Out1 : Outport
  wires:
  Extract Bits1/1 -> Data Type Conversion8/1
  In1/1 -> Extract Bits1/1
  Data Type Conversion8/1 -> Out1/1

== system D53_LKA_Software/LL/LLOn/LKA/Lane Following (LF)/Trajectory Following Control (TFC)/Feedback Control (FbCtl)/Subsystem/Signal Latching2/if action  ==
  In : Inport
  Action Port : ActionPort  InitializeStates=reset
  Out : Outport
  wires:
  In/1 -> Out/1

== system D53_LKA_Software/LL/LLOn/LKA/Plan To LaneFollowing (PTLF)/InsideJudge1/If Action Subsystem/If Action Subsystem/Signal Latching/if action  ==
  In : Inport
  Action Port : ActionPort
  Out : Outport
  wires:
  In/1 -> Out/1

== system D53_LKA_Software/LL/LLOn/LKA/Plan To LaneFollowing (PTLF)/InsideJudge1/If Action Subsystem/If Action Subsystem/Signal Latching1/if action  ==
  In : Inport
  Action Port : ActionPort
  Out : Outport
  wires:
  In/1 -> Out/1

== system D53_LKA_Software/LL/LLOn/LKA/Plan To LaneFollowing (PTLF)/InsideJudge1/If Action Subsystem1/If Action Subsystem/Signal Latching/if action  ==
  In : Inport
  Action Port : ActionPort
  Out : Outport
  wires:
  In/1 -> Out/1

== system D53_LKA_Software/LL/LLOn/LKA/Plan To LaneFollowing (PTLF)/InsideJudge1/If Action Subsystem1/If Action Subsystem/Signal Latching1/if action  ==
  In : Inport
  Action Port : ActionPort
  Out : Outport
  wires:
  In/1 -> Out/1

== system D53_LKA_Software/LL/LLOn/LL State Determination (LLStateDet)/LL State Machine Conditions (LLSMCon)/Activation Condition (ActvC)/Deviation Threshold Condition (DvtThresCon)/Deviation Threshold Judgement LDW (DvtThresJdg)/Deviation Speed Detection (DvtSpdDet)/Ph1SWA ==
  Action Port : ActionPort  InitializeStates=reset
  Constant : Constant  OutDataTypeStr=single
  Out : Outport
  wires:
  Constant/1 -> Out/1

== system D53_LKA_Software/LL/LLOn/LL State Determination (LLStateDet)/LL State Machine Conditions (LLSMCon)/Activation Condition (ActvC)/Deviation Threshold Condition (DvtThresCon)/Deviation Threshold Judgement LDW (DvtThresJdg)/Deviation Speed Detection (DvtSpdDet)/Ph2SWA ==
  Action Port : ActionPort  InitializeStates=reset
  Constant : Constant  Value=-1  OutDataTypeStr=single
  Out : Outport
  wires:
  Constant/1 -> Out/1

== system D53_LKA_Software/LL/LLOn/LL State Determination (LLStateDet)/LL State Machine Conditions (LLSMCon)/Activation Condition (ActvC)/Deviation Threshold Condition (DvtThresCon)/Deviation Threshold Judgement LDW (DvtThresJdg)/Deviation Speed Detection (DvtSpdDet)/Ph3SWA ==
  Action Port : ActionPort  InitializeStates=reset
  Constant : Constant  Value=0  OutDataTypeStr=single
  Out : Outport
  wires:
  Constant/1 -> Out/1

== system D53_LKA_Software/LL/LLOn/LL State Determination (LLStateDet)/LL State Machine Conditions (LLSMCon)/Activation Condition (ActvC)/Deviation Threshold Condition (DvtThresCon)/Deviation Threshold Judgement LKA (DvtThresJdg)/Deviation Speed Detection (DvtSpdDet)/Ph1SWA ==
  Action Port : ActionPort  InitializeStates=reset
  Constant : Constant  OutDataTypeStr=single
  Out : Outport
  wires:
  Constant/1 -> Out/1

== system D53_LKA_Software/LL/LLOn/LL State Determination (LLStateDet)/LL State Machine Conditions (LLSMCon)/Activation Condition (ActvC)/Deviation Threshold Condition (DvtThresCon)/Deviation Threshold Judgement LKA (DvtThresJdg)/Deviation Speed Detection (DvtSpdDet)/Ph2SWA ==
  Action Port : ActionPort  InitializeStates=reset
  Constant : Constant  Value=-1  OutDataTypeStr=single
  Out : Outport
  wires:
  Constant/1 -> Out/1

== system D53_LKA_Software/LL/LLOn/LL State Determination (LLStateDet)/LL State Machine Conditions (LLSMCon)/Activation Condition (ActvC)/Deviation Threshold Condition (DvtThresCon)/Deviation Threshold Judgement LKA (DvtThresJdg)/Deviation Speed Detection (DvtSpdDet)/Ph3SWA ==
  Action Port : ActionPort  InitializeStates=reset
  Constant : Constant  Value=0  OutDataTypeStr=single
  Out : Outport
  wires:
  Constant/1 -> Out/1

== system D53_LKA_Software/LL/LLOn/LL State Determination (LLStateDet)/LL State Machine Conditions (LLSMCon)/Deactivation Condition (DeactvC)/Deviation Threshold Condition (DvtThresCon)/Deviation Threshold Judgement LDW (DvtThresJdg)/Deviation Speed Detection (DvtSpdDet)/Ph1SWA ==
  Action Port : ActionPort  InitializeStates=reset
  Constant : Constant  OutDataTypeStr=single
  Out : Outport
  wires:
  Constant/1 -> Out/1

== system D53_LKA_Software/LL/LLOn/LL State Determination (LLStateDet)/LL State Machine Conditions (LLSMCon)/Deactivation Condition (DeactvC)/Deviation Threshold Condition (DvtThresCon)/Deviation Threshold Judgement LDW (DvtThresJdg)/Deviation Speed Detection (DvtSpdDet)/Ph2SWA ==
  Action Port : ActionPort  InitializeStates=reset
  Constant : Constant  Value=-1  OutDataTypeStr=single
  Out : Outport
  wires:
  Constant/1 -> Out/1

== system D53_LKA_Software/LL/LLOn/LL State Determination (LLStateDet)/LL State Machine Conditions (LLSMCon)/Deactivation Condition (DeactvC)/Deviation Threshold Condition (DvtThresCon)/Deviation Threshold Judgement LDW (DvtThresJdg)/Deviation Speed Detection (DvtSpdDet)/Ph3SWA ==
  Action Port : ActionPort  InitializeStates=reset
  Constant : Constant  Value=0  OutDataTypeStr=single
  Out : Outport
  wires:
  Constant/1 -> Out/1

== system D53_LKA_Software/LL/LLOn/LL State Determination (LLStateDet)/LL State Machine Conditions (LLSMCon)/Deactivation Condition (DeactvC)/Deviation Threshold Condition (DvtThresCon)/Deviation Threshold Judgement LKA (DvtThresJdg)/Deviation Speed Detection (DvtSpdDet)/Ph1SWA ==
  Action Port : ActionPort  InitializeStates=reset
  Constant : Constant  OutDataTypeStr=single
  Out : Outport
  wires:
  Constant/1 -> Out/1

== system D53_LKA_Software/LL/LLOn/LL State Determination (LLStateDet)/LL State Machine Conditions (LLSMCon)/Deactivation Condition (DeactvC)/Deviation Threshold Condition (DvtThresCon)/Deviation Threshold Judgement LKA (DvtThresJdg)/Deviation Speed Detection (DvtSpdDet)/Ph2SWA ==
  Action Port : ActionPort  InitializeStates=reset
  Constant : Constant  Value=-1  OutDataTypeStr=single
  Out : Outport
  wires:
  Constant/1 -> Out/1

== system D53_LKA_Software/LL/LLOn/LL State Determination (LLStateDet)/LL State Machine Conditions (LLSMCon)/Deactivation Condition (DeactvC)/Deviation Threshold Condition (DvtThresCon)/Deviation Threshold Judgement LKA (DvtThresJdg)/Deviation Speed Detection (DvtSpdDet)/Ph3SWA ==
  Action Port : ActionPort  InitializeStates=reset
  Constant : Constant  Value=0  OutDataTypeStr=single
  Out : Outport
  wires:
  Constant/1 -> Out/1

== system D53_LKA_Software/LL/LLOn/LL State Determination (LLStateDet)/LL State Machine Conditions (LLSMCon)/Disable Condition (DisblC)/Driver Intent Condition (DrvInttC)/Take-Over Steering Check (TkOvStChk)/Time Delay (TDel)/If Action Subsystem ==
  Action Port : ActionPort  InitializeStates=reset
  Constant : Constant  OutDataTypeStr=boolean  SampleTime=-1
  Out : Outport
  wires:
  Constant/1 -> Out/1

== system D53_LKA_Software/LL/LLOn/LL State Determination (LLStateDet)/LL State Machine Conditions (LLSMCon)/Disable Condition (DisblC)/Driver Intent Condition (DrvInttC)/Take-Over Steering Check (TkOvStChk)/Time Delay (TDel)/If Action Subsystem1 ==
  Action Port : ActionPort  InitializeStates=reset
  Constant : Constant  Value=0  OutDataTypeStr=boolean  SampleTime=-1
  Out : Outport
  wires:
  Constant/1 -> Out/1

== system D53_LKA_Software/LL/LLOn/LL State Determination (LLStateDet)/LL State Machine Conditions (LLSMCon)/Disable Condition (DisblC)/Driver Intent Condition (DrvInttC)/Take-Over Steering Check (TkOvStChk)/Time Delay (TDel)/If Action Subsystem3 ==
  In1 : Inport
  Action Port : ActionPort  InitializeStates=reset
  Out : Outport
  wires:
  In1/1 -> Out/1

== system D53_LKA_Software/LL/LLOn/LL State Determination (LLStateDet)/LL State Machine Conditions (LLSMCon)/Disable Condition (DisblC)/Driver Intent Condition (DrvInttC)/Take-Over Steering Check (TkOvStChk)/Time Delay (TDel)/Sum Condition1 ==
  In : Inport
  Sum : Inport  Port=2
  state = reset : EnablePort  StatesWhenEnabling=reset
  Add1 : Sum  OutDataTypeStr=uint16
  Memory : Memory  InheritSampleTime=on
  Relational Operator : RelationalOperator  Operator=<=  OutDataTypeStr=boolean  RndMeth=Nearest
  Saturation : Saturate  UpperLimit=10000  LowerLimit=0
  Out : Outport  OutputWhenDisabled=reset  InitialOutput=0
  wires:
  Memory/1 -> Add1/2
  Add1/1 -> Saturation/1
  In/1 -> Add1/1
  Sum/1 -> Relational Operator/2
  Relational Operator/1 -> Out/1
  Saturation/1 -> Memory/1, Relational Operator/1

== matlab function D53_LKA_Software/LL/Human Machine Interface (HMI)/HMI_Popup_Status ==
  data: HMI_Popup_Status output; stDACmode input; LKA_STATE input; HandsOff input; camera_common_fault input; Front_Camera_Blocked input; stFaultCSyn input
function HMI_Popup_Status = fcn(stDACmode,LKA_STATE,HandsOff,camera_common_fault,Front_Camera_Blocked,stFaultCSyn)
if stDACmode==2&&LKA_STATE==6 %车道保持辅助故障
    HMI_Popup_Status=uint8(6);
elseif stDACmode==2&&camera_common_fault==1&&Front_Camera_Blocked~=5  %车道保持辅助暂不可用
    HMI_Popup_Status=uint8(3);
elseif (stDACmode==2||stDACmode==1)&&(Front_Camera_Blocked==5)   %摄像头被遮挡
    HMI_Popup_Status=uint8(4);
elseif (stDACmode==2||stDACmode==1)&&HandsOff==1  %手握方向盘
    HMI_Popup_Status=uint8(2);    
elseif stDACmode==2&&(LKA_STATE==2)
    HMI_Popup_Status=uint8(1);
elseif stDACmode~=2&&stFaultCSyn==0
    HMI_Popup_Status=uint8(8);
elseif stFaultCSyn==0
    HMI_Popup_Status=uint8(7);
elseif stDACmode==2&&(LKA_STATE==0||LKA_STATE==1)
    HMI_Popup_Status=uint8(0);
else
    HMI_Popup_Status=uint8(0);
end

== matlab function D53_LKA_Software/LL/Human Machine Interface (HMI)/Hands_off_warning ==
  data: Hands_off_warning output; HandsOff input
function Hands_off_warning = fcn(HandsOff)
Hands_off_warning = uint8(0);
if HandsOff==0
    Hands_off_warning= uint8(0);
elseif HandsOff==1
    Hands_off_warning= uint8(1);
else
    Hands_off_warning= uint8(0);
end

== matlab function D53_LKA_Software/LL/Human Machine Interface (HMI)/LDW_Flag ==
  data: HMI_stDACmode input; HMI_LKA_STATE input; LDW_Flag output; HMI_LDWWarnInfo input
function LDW_Flag = fcn(HMI_stDACmode, HMI_LKA_STATE, HMI_LDWWarnInfo)
if HMI_stDACmode==1
    LDW_Flag = uint8(0);
    if HMI_LDWWarnInfo==1
        LDW_Flag=uint8(1);
    elseif HMI_LDWWarnInfo==2
        LDW_Flag=uint8(2);
    else
        LDW_Flag=uint8(0);
    end
elseif HMI_stDACmode==2
    LDW_Flag = uint8(0);
    if HMI_LDWWarnInfo==1 && HMI_LKA_STATE==4
        LDW_Flag=uint8(1);
    elseif HMI_LDWWarnInfo==2 && HMI_LKA_STATE==5
        LDW_Flag=uint8(2);
    else
        LDW_Flag=uint8(0);
    end    
else
    LDW_Flag=uint8(0);
end
end

== matlab function D53_LKA_Software/LL/Human Machine Interface (HMI)/LDW_Status_Display ==
  data: stDACmode input; LDW_Status_Display output; LDW_STATE input
function LDW_Status_Display = fcn(stDACmode,LDW_STATE)
if (stDACmode==1)&&LDW_STATE~=6
    LDW_Status_Display=uint8(1);
elseif (stDACmode==1)&&LDW_STATE==6
    LDW_Status_Display=uint8(2);
else
    LDW_Status_Display=uint8(0);
end

== matlab function D53_LKA_Software/LL/Human Machine Interface (HMI)/LKA_Status_Display ==
  data: stDACmode input; LKA_Status_Display output; LKA_STATE input
function LKA_Status_Display  = fcn(stDACmode,LKA_STATE)
LKA_Status_Display = single(0);
if stDACmode==2&&LKA_STATE~=6
    LKA_Status_Display=single(1);
elseif stDACmode==2&&LKA_STATE==6
    LKA_Status_Display=single(2);
else
    LKA_Status_Display=single(0);
end

== matlab function D53_LKA_Software/LL/Human Machine Interface (HMI)/LKA_action_indication ==
  data: LKA_action_indication output; stDACmode input; LKA_STATE input
function LKA_action_indication = fcn(stDACmode,LKA_STATE)
if stDACmode==2&&LKA_STATE==2
    LKA_action_indication=uint8(1);
elseif stDACmode==2&&LKA_STATE==3
    LKA_action_indication=uint8(2);
elseif stDACmode==2&&(LKA_STATE==4||LKA_STATE==5)
    LKA_action_indication=uint8(3);
else
    LKA_action_indication=uint8(0);
end
